simulink model "UseCase_v5"  (R2024b)
settings: Solver=ode1  StartTime=0.0  StopTime=365*24  FixedStep=0.2  RelTol=1e-3
libraries: filter_lib x5, Harvester_lib x3, buffer_lib x3, Demand_lib x2, storage_lib x2, transport_lib x1
settings Model: SimulationMode=accelerator  Creator=marcv  LastModifiedBy=20223126
settings RTWCC: GPUComputeCapability=3.5

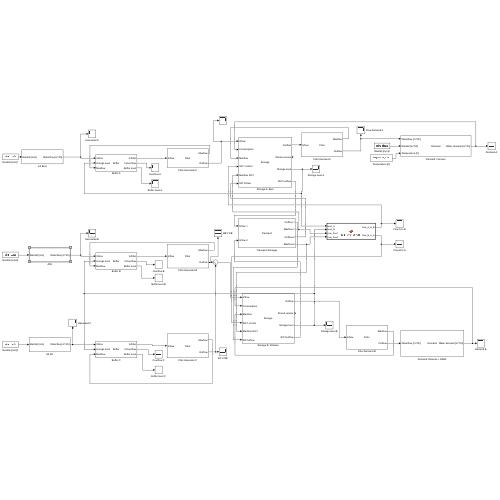
[thumbnail: Simulink's stored preview of the top-level diagram]
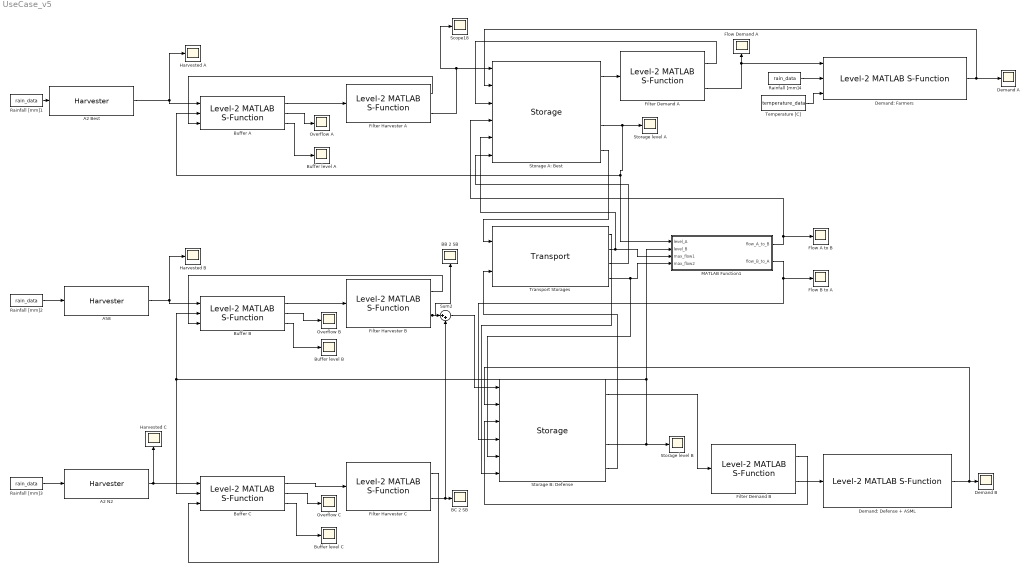
== system UseCase_v5 ==
  A2 Best : Harvester_lib/Harvester  Type_harvester=Dependant on ground water (tunnel)  inflow_groundwater=91  Area=64000
  A2 N2 : Harvester_lib/Harvester  Type_harvester=Independant on ground water (resevoir, road ect.)  inflow_groundwater=1  Area=21e4
  A58 : Harvester_lib/Harvester  Type_harvester=Independant on ground water (resevoir, road ect.)  inflow_groundwater=1  Area=13.5e4
  BB 2 SB : Scope
  BC 2 SB : Scope
  Buffer A : buffer_lib/Level-2 MATLAB S-Function  Parameter1=2e4
  Buffer B : buffer_lib/Level-2 MATLAB S-Function  Parameter1=7e3
  Buffer C : buffer_lib/Level-2 MATLAB S-Function  Parameter1=1e4
  Buffer level A : Scope
  Buffer level B : Scope
  Buffer level C : Scope
  Demand A : Scope
  Demand B : Scope
  Demand: Defense + ASML : Demand_lib/Level-2 MATLAB S-Function  Type_demand=Constant demand  Constant_demand=7e5  Crop_type=Potato  Area=8.5e5  Type_soil=Clay soil  Type_control=Normal control  Predictive_steps=5
  Demand: Farmers : Demand_lib/Level-2 MATLAB S-Function  Type_demand=Agriculture  Constant_demand=6e5  Crop_type=Potato  Area=5e5  Type_soil=Clay soil  Type_control=Normal control  Predictive_steps=5
  Filter Demand A : filter_lib/Level-2 MATLAB S-Function  filteroption=Custom filter  Parameter4=Cyclone-sand-UV [90 m3/h]  Parameter1=400  Parameter2=1
  Filter Demand B : filter_lib/Level-2 MATLAB S-Function  filteroption=Custom filter  Parameter4=Cyclone-sand-UV [90 m3/h]  Parameter1=100  Parameter2=1
  Filter Harvester A : filter_lib/Level-2 MATLAB S-Function  filteroption=Custom filter  Parameter4=Cyclone-sand-UV [90 m3/h]  Parameter1=200  Parameter2=1
  Filter Harvester B : filter_lib/Level-2 MATLAB S-Function  filteroption=Custom filter  Parameter4=Cyclone-sand-UV [90 m3/h]  Parameter1=100  Parameter2=1
  Filter Harvester C : filter_lib/Level-2 MATLAB S-Function  filteroption=Custom filter  Parameter4=Cyclone-sand-UV [90 m3/h]  Parameter1=100  Parameter2=1
  Flow A to B : Scope
  Flow B to A : Scope
  Flow Demand A : Scope
  Harvested A : Scope
  Harvested B : Scope
  Harvested C : Scope
  MATLAB Function1 : MATLAB Function  TreatAsAtomicUnit=on
  Overflow A : Scope
  Overflow B : Scope
  Overflow C : Scope
  Rainfall [mm]{1..4} (4 alike) : FromWorkspace  VariableName=rain_data  OutDataTypeStr=double  SampleTime=1
  Scope18 : Scope
  Storage A: Best : storage_lib/Storage  Parameter1=8e4 %10e4  Parameter2=0.65  Parameter3=1 interconnection
  Storage B: Defense : storage_lib/Storage  Parameter1=22.5e4  Parameter2=0.7  Parameter3=1 interconnection
  Storage level A : Scope
  Storage level B : Scope
  Sum2 : Sum  Inputs=|++
  Temperature [C] : FromWorkspace  VariableName=temperature_data  OutDataTypeStr=double  SampleTime=1
  Transport Storages : transport_lib/Transport  max_flow_result1=200  max_flow_result2=200  flowDirec=Bidirectional  setupopt=Transport only  Transporttype=Custom  Dist=210  elevation=1  width=1  depth=1  diameter=1  dP=2  customflow=200  filteroption=Common filter  Fflowmax=0  dPfilter=0  selectedfilter=Sand [90 m3/h (UDI 4U4604)]  filterparallel=1
  wires:
  Rainfall [mm]1/1 -> A2 Best/1
  A2 Best/1 -> Buffer A/1, Harvested A/1
  Buffer A/3 -> Buffer level A/1
  Filter Harvester A/1 -> Buffer A/3
  Buffer A/1 -> Filter Harvester A/1
  Buffer A/2 -> Overflow A/1
  Filter Harvester A/2 -> Storage A: Best/1, Scope18/1
  Storage A: Best/1 -> Filter Demand A/1
  Storage A: Best/3 -> Buffer A/2, MATLAB Function1/1(level_A), Storage level A/1
  Storage B: Defense/3 -> Storage level B/1, MATLAB Function1/2(level_B), Buffer C/2, Buffer B/2
  Buffer B/2 -> Overflow B/1
  Buffer B/1 -> Filter Harvester B/1
  Filter Harvester B/1 -> Buffer B/3
  A58/1 -> Buffer B/1, Harvested B/1
  Buffer B/3 -> Buffer level B/1
  Rainfall [mm]2/1 -> A58/1
  Demand: Farmers/1 -> Storage A: Best/2, Demand A/1
  Demand: Defense + ASML/1 -> Demand B/1, Storage B: Defense/2
  Storage B: Defense/1 -> Filter Demand B/1
  Rainfall [mm]4/1 -> Demand: Farmers/2
  Filter Harvester C/1 -> Buffer C/3
  Buffer C/2 -> Overflow C/1
  Rainfall [mm]3/1 -> A2 N2/1
  Buffer C/1 -> Filter Harvester C/1
  Buffer C/3 -> Buffer level C/1
  A2 N2/1 -> Buffer C/1, Harvested C/1
  Filter Harvester B/2 -> BB 2 SB/1, Sum2/1
  Sum2/1 -> Storage B: Defense/1
  Filter Harvester C/2 -> BC 2 SB/1, Sum2/2
  Filter Demand A/1 -> Storage A: Best/3
  Filter Demand A/2 -> Flow Demand A/1, Demand: Farmers/1
  Filter Demand B/2 -> Demand: Defense + ASML/1
  Filter Demand B/1 -> Storage B: Defense/3
  Transport Storages/2 -> Storage A: Best/5, MATLAB Function1/3(max_flow1)
  Transport Storages/4 -> Storage B: Defense/5, MATLAB Function1/4(max_flow2)
  MATLAB Function1/1(flow_A_to_B) -> Storage A: Best/4, Flow A to B/1
  Storage A: Best/4 -> Transport Storages/1
  Transport Storages/1 -> Storage B: Defense/6
  MATLAB Function1/2(flow_B_to_A) -> Storage B: Defense/4, Flow B to A/1
  Storage B: Defense/4 -> Transport Storages/2
  Transport Storages/3 -> Storage A: Best/6
  Temperature [C]/1 -> Demand: Farmers/3

== matlab function UseCase_v5/MATLAB Function1 ==
  data: level_A input; flow_A_to_B output; level_B input; max_flow1 input; max_flow2 input; flow_B_to_A output
function [flow_A_to_B, flow_B_to_A] = real_time_control(level_A, level_B, max_flow1, max_flow2)

thresholdA = 0.05;
thresholdB = 0.05;

% min_threshold = 0;
flow_A_to_B = 0;
flow_B_to_A = 0;
gain = 5;

% Flow from A to B
if (level_A > level_B) && (level_A > thresholdA)
    flow_A_to_B = min(gain*(level_A - level_B), 1) * max_flow1;


% Flow from B to A
elseif (level_B > level_A) && (level_B > thresholdB)
    flow_B_to_A = min(gain*(level_B - level_A), 1) * max_flow2;

% elseif (level_A > level_B) && (level_B < min_threshold)
%     flow_A_to_B = min((level_A - level_B), 1) * max_flow1;
% 
% elseif (level_B > level_A) && (level_A < min_threshold)
%     flow_B_to_A = min((level_B - level_A), 1) * max_flow2;


end
